simulink model "calc_pid_speed_x"  (R2020a)
settings: Solver=VariableStepAuto  StartTime=0.0  StopTime=5  RelTol=1e-3
libraries: checkpacklib x1
settings Model: Creator=Tamer  LastModifiedBy=Tamer

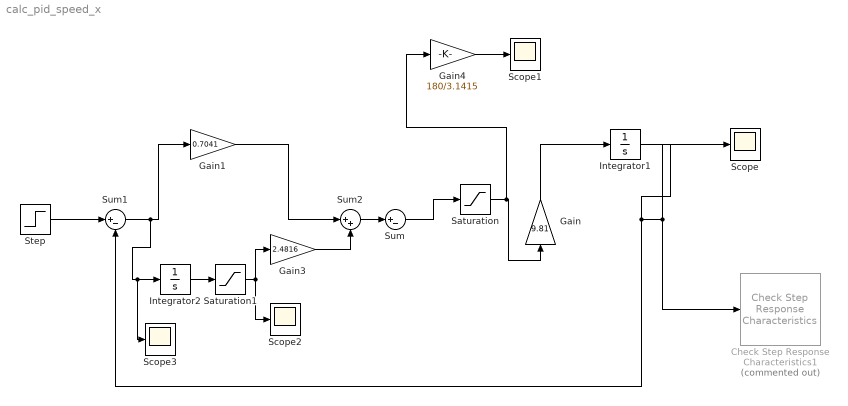
== system calc_pid_speed_x ==
  Check Step Response Characteristics1 : checkpacklib/Check Step Response  Characteristics  Commented=on  InstantiateOnLoad=on  enabled=on  stopWhenAssertionFail=off  export=off  ViewDlgPos=[]  OpenViewOnLoad=off  LaunchViewOnOpen=off  TimeUnits=seconds  EnableStepResponseBound=on  InitialValue=0  FinalValue=1  StepTime=0  RiseTime=1  PercentRise=80  SettlingTime=1.1  PercentSettling=1  PercentOvershoot=10  PercentUndershoot=1
      settings: SourceProductBaseCode=CT,ID,MT,SO
  Gain : Gain  Gain=9.81
  Gain1 : Gain  Gain=0.7041
  Gain3 : Gain  Gain=2.4816
  Gain4 : Gain  Gain=180/3.1415
  Integrator1 : Integrator
  Integrator2 : Integrator
  Saturation : Saturate  UpperLimit=deg2rad(50)  LowerLimit=-deg2rad(50)  ZeroCross=off
  Saturation1 : Saturate  UpperLimit=5  LowerLimit=-5
  Scope{,1..3} (4 alike) : Scope
  Step : Step  Time=0  After=3  SampleTime=0
  Sum : Sum  Inputs=|+-
  Sum1 : Sum  Inputs=|+-
  Sum2 : Sum  Inputs=|++
  wires:
  Gain/1 -> Integrator1/1
  Integrator1/1 -> Sum1/2, Check Step Response Characteristics1/1, Scope/1
  Gain1/1 -> Sum2/1
  Sum2/1 -> Sum/1
  Gain3/1 -> Sum2/2
  Step/1 -> Sum1/1
  Gain4/1 -> Scope1/1
  Saturation/1 -> Gain4/1, Gain/1
  Sum/1 -> Saturation/1
  Sum1/1 -> Scope3/1, Integrator2/1, Gain1/1
  Integrator2/1 -> Saturation1/1
  Saturation1/1 -> Gain3/1, Scope2/1
